simulink model "BufMinMax_tests"  (R2024a)
settings: Solver=VariableStepAuto  StartTime=0.0  StopTime=2  RelTol=1e-3
undefined symbols (not defined in the file or in its folder): BUFFER_LEN
settings Model: Creator=Jan Rosa  LastModifiedBy=Jan Rosa

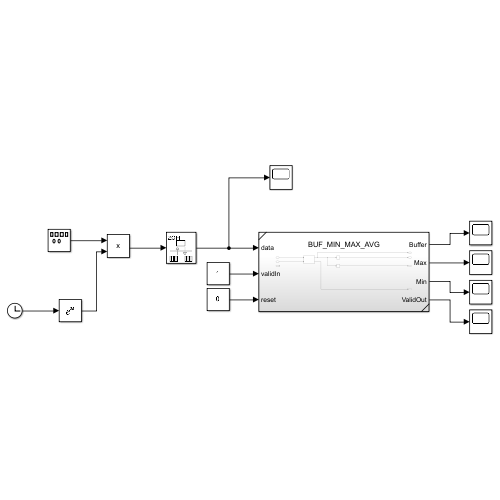
[thumbnail: Simulink's stored preview of the top-level diagram]
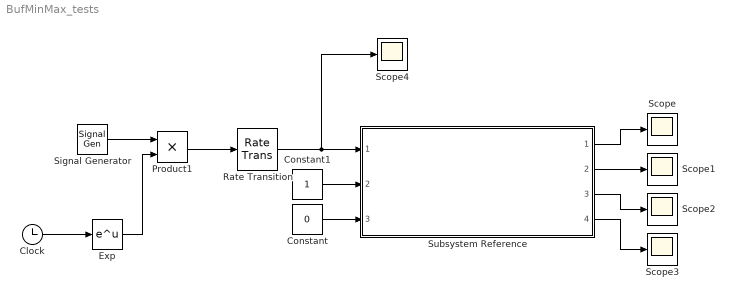
== system BufMinMax_tests ==
  Clock : Clock
  Constant : Constant  Value=0  OutDataTypeStr=boolean
  Constant1 : Constant  OutDataTypeStr=boolean
  Exp : Math
  Product1 : Product
  Rate Transition : RateTransition  OutPortSampleTime=1/BUFFER_LEN
  Scope{,1..4} (5 alike) : Scope
  Signal Generator : SignalGenerator  Frequency=50
  Subsystem Reference : Subsystem  ReferencedSubsystem=BUF_MIN_MAX_AVG
  wires:
  Product1/1 -> Rate Transition/1
  Rate Transition/1 -> Scope4/1, Subsystem Reference/1
  Constant1/1 -> Subsystem Reference/2
  Constant/1 -> Subsystem Reference/3
  Subsystem Reference/1 -> Scope/1
  Subsystem Reference/4 -> Scope3/1
  Subsystem Reference/3 -> Scope2/1
  Subsystem Reference/2 -> Scope1/1
  Clock/1 -> Exp/1
  Exp/1 -> Product1/2
  Signal Generator/1 -> Product1/1
